simulink model "Simulink_es2_tesina"  (R2022b)
settings: Solver=VariableStepAuto  StartTime=0.0  StopTime=10.0  RelTol=1e-3
libraries: cstblocks x2
settings Model: Creator=criss  LastModifiedBy=criss

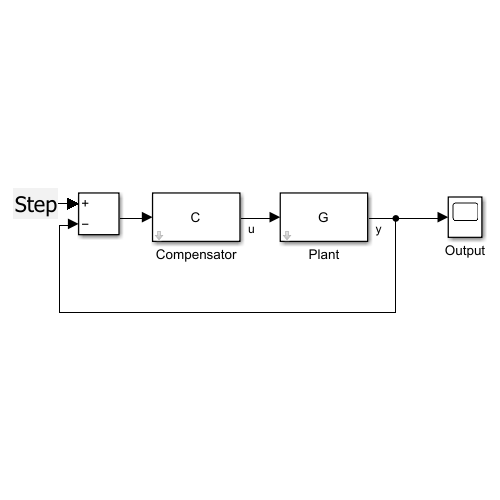
[thumbnail: Simulink's stored preview of the top-level diagram]
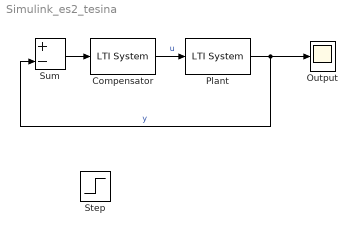
== system Simulink_es2_tesina ==
  Compensator : cstblocks/LTI System  sys=C  IC=[]
  Output : Scope
  Plant : cstblocks/LTI System  sys=G  IC=[]
  Sum : Sum  Inputs=+-
  Step : Step  IOType=siggen  Time=0  SampleTime=0
  wires:
  Sum/1 -> Compensator/1
  Compensator/1 -> Plant/1  "u"
  Plant/1 -> Sum/2, Output/1  "y"
